simulink model "Integration_1.0"  (R2024b)
settings: Solver=VariableStepAuto  StartTime=0.0  StopTime=4  RelTol=1e-3
undefined symbols (not defined in the file): Ion, Lithium, Ts_Control
libraries: spsSeriesRLCBranchLib x37, ee_lib x30, nesl_utility x24, simulink x23, slpidlib x21, spsCurrentVoltageSimscapeInterfaceLib x18, powerlib_extras x18, spsThreePhaseVIMeasurementLib x7, spsThreePhaseSeriesRLCBranchLib x7, spsGroundLib x7, spsPWMGeneratorDCDCLib x6, spsPVArrayLib x6
(part 1 of 5)
settings Model: Creator=DELL  LastModifiedBy=mitphanase

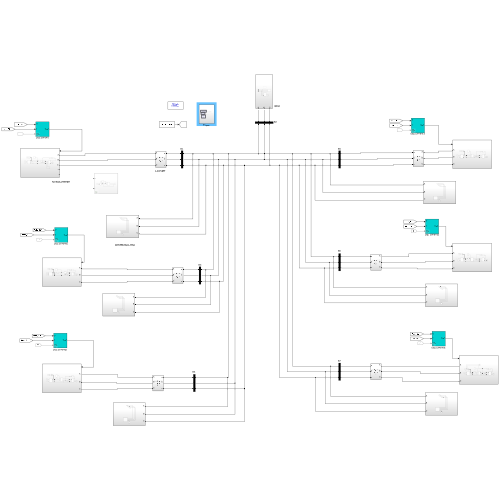
[thumbnail: Simulink's stored preview of the top-level diagram]
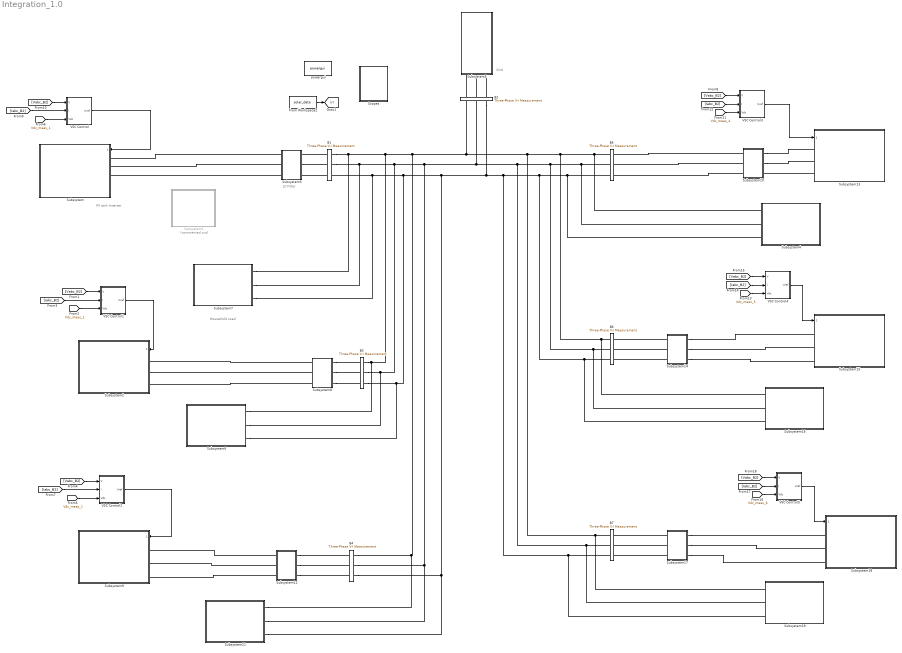
== system Integration_1.0 ==
  note: Household Load
  note: LC Filter
  note: Grid
  note: PV with Inverter
  B1 : spsThreePhaseVIMeasurementLib/Three-Phase V-I Measurement  VoltageMeasurement=phase-to-phase  SetLabelV=on  LabelV=Vabc_B1  Vpu=off  VpuLL=off  CurrentMeasurement=yes  SetLabelI=on  LabelI=Iabc_B1  Ipu=off  Pbase=100e6  Vbase=1000  OutputType=Magnitude  PhasorSimulation=off  PSBequivalent=0
  B2 : spsThreePhaseVIMeasurementLib/Three-Phase V-I Measurement  VoltageMeasurement=phase-to-phase  SetLabelV=on  LabelV=Vabc_B2  Vpu=off  VpuLL=off  CurrentMeasurement=yes  SetLabelI=on  LabelI=Iabc_B2  Ipu=off  Pbase=100e6  Vbase=500e3  OutputType=Magnitude  PhasorSimulation=off  PSBequivalent=0
  B3 : spsThreePhaseVIMeasurementLib/Three-Phase V-I Measurement  VoltageMeasurement=phase-to-phase  SetLabelV=on  LabelV=Vabc_B3  Vpu=off  VpuLL=off  CurrentMeasurement=yes  SetLabelI=on  LabelI=Iabc_B3  Ipu=off  Pbase=100e6  Vbase=1000  OutputType=Magnitude  PhasorSimulation=off  PSBequivalent=0
  B4 : spsThreePhaseVIMeasurementLib/Three-Phase V-I Measurement  VoltageMeasurement=phase-to-phase  SetLabelV=on  LabelV=Vabc_B4  Vpu=off  VpuLL=off  CurrentMeasurement=yes  SetLabelI=on  LabelI=Iabc_B4  Ipu=off  Pbase=100e6  Vbase=1000  OutputType=Magnitude  PhasorSimulation=off  PSBequivalent=0
  B5 : spsThreePhaseVIMeasurementLib/Three-Phase V-I Measurement  VoltageMeasurement=phase-to-phase  SetLabelV=on  LabelV=Vabc_B5  Vpu=off  VpuLL=off  CurrentMeasurement=yes  SetLabelI=on  LabelI=Iabc_B5  Ipu=off  Pbase=100e6  Vbase=1000  OutputType=Magnitude  PhasorSimulation=off  PSBequivalent=0
  B6 : spsThreePhaseVIMeasurementLib/Three-Phase V-I Measurement  VoltageMeasurement=phase-to-phase  SetLabelV=on  LabelV=Vabc_B6  Vpu=off  VpuLL=off  CurrentMeasurement=yes  SetLabelI=on  LabelI=Iabc_B6  Ipu=off  Pbase=100e6  Vbase=1000  OutputType=Magnitude  PhasorSimulation=off  PSBequivalent=0
  B7 : spsThreePhaseVIMeasurementLib/Three-Phase V-I Measurement  VoltageMeasurement=phase-to-phase  SetLabelV=on  LabelV=Vabc_B7  Vpu=off  VpuLL=off  CurrentMeasurement=yes  SetLabelI=on  LabelI=Iabc_B7  Ipu=off  Pbase=100e6  Vbase=1000  OutputType=Magnitude  PhasorSimulation=off  PSBequivalent=0
  From Workspace2 : FromWorkspace  VariableName=solar_data  OutDataTypeStr=double  SampleTime=0.01
  Scopes : Subsystem
  Subsystem : Subsystem
  Subsystem1 : Subsystem  Commented=on
  Subsystem10 : Subsystem
  Subsystem11 : Subsystem
  Subsystem12 : Subsystem
  Subsystem13 : Subsystem
  Subsystem14 : Subsystem
  Subsystem15 : Subsystem
  Subsystem16 : Subsystem
  Subsystem17 : Subsystem
  Subsystem18 : Subsystem
  Subsystem19 : Subsystem
  Subsystem2 : Subsystem
  Subsystem3 : Subsystem
  Subsystem4 : Subsystem
  Subsystem5 : Subsystem
  Subsystem6 : Subsystem
  Subsystem7 : Subsystem
  Subsystem8 : Subsystem
  Subsystem9 : Subsystem
  VSC Control : Subsystem  mask(VSC Main Controller){nom=[ 17e3  50 ], Vnom=[ 400 400 ], Vnom_dc=600, RLxfo=[0  0 ], RLchoke=[0  0  ], K_VDCreg=[18  600], K_Ireg=[0.2 20], Ts=Ts_Control}
      mask prompts: nom "Nominal power and frequency [ Pnom(VA)  Fnom(Hz) ]:"; Vnom "Nominal primary and secondary voltages (Vrms LL) [ Vnom_prim   Vnom_sec ]:"; Vnom_dc "Nominal DC bus voltage (V):"; RLxfo "Total transformer leakage impedance (pu/Pnom) [ Rxfo  Lxf ]"; RLchoke "Choke impedance [ R(ohm) L(H) ]"; K_VDCreg "VDC regultator gains [ Kp  Ki ]:"; K_Ireg "Current regulator gains [ Kp  Ki ]:"; Ts "Sample time"
      mask init:
      | Pnom=nom(1);
      | Fnom=nom(2);
      | Vnom_prim=Vnom(1);
      | Vnom_sec=Vnom(2);
      | Zbase=Vnom_sec^2/Pnom;
      | Rtot_pu=RLxfo(1) + RLchoke(1)/Zbase;
      | Ltot_pu=RLxfo(2) + RLchoke(2)/(Zbase/(2*pi*Fnom));
      | Kp_VDCreg=K_VDCreg(1);
      | Ki_VDCreg=K_VDCreg(2);
      | Kp_Ireg=K_Ireg(1);
      | Ki_Ireg=K_Ireg(2);
      | Vdc_ref=Vnom_dc;
  VSC Control1 : Subsystem  mask(VSC Main Controller){nom=[ 5e3  50 ], Vnom=[ 400 400 ], Vnom_dc=600, RLxfo=[0  0 ], RLchoke=[0  0  ], K_VDCreg=[18  600], K_Ireg=[0.2 20], Ts=Ts_Control}
      mask prompts: nom "Nominal power and frequency [ Pnom(VA)  Fnom(Hz) ]:"; Vnom "Nominal primary and secondary voltages (Vrms LL) [ Vnom_prim   Vnom_sec ]:"; Vnom_dc "Nominal DC bus voltage (V):"; RLxfo "Total transformer leakage impedance (pu/Pnom) [ Rxfo  Lxf ]"; RLchoke "Choke impedance [ R(ohm) L(H) ]"; K_VDCreg "VDC regultator gains [ Kp  Ki ]:"; K_Ireg "Current regulator gains [ Kp  Ki ]:"; Ts "Sample time"
      mask init: same as Integration_1.0/VSC Control
  VSC Control2 : Subsystem  mask(VSC Main Controller){nom=[ 5e3  50 ], Vnom=[ 400 400 ], Vnom_dc=600, RLxfo=[0  0 ], RLchoke=[0  0  ], K_VDCreg=[18  600], K_Ireg=[0.2 20], Ts=Ts_Control}
      mask prompts: nom "Nominal power and frequency [ Pnom(VA)  Fnom(Hz) ]:"; Vnom "Nominal primary and secondary voltages (Vrms LL) [ Vnom_prim   Vnom_sec ]:"; Vnom_dc "Nominal DC bus voltage (V):"; RLxfo "Total transformer leakage impedance (pu/Pnom) [ Rxfo  Lxf ]"; RLchoke "Choke impedance [ R(ohm) L(H) ]"; K_VDCreg "VDC regultator gains [ Kp  Ki ]:"; K_Ireg "Current regulator gains [ Kp  Ki ]:"; Ts "Sample time"
      mask init: same as Integration_1.0/VSC Control
  VSC Control3 : Subsystem  mask(VSC Main Controller){nom=[ 12.5e3  50 ], Vnom=[ 400 400 ], Vnom_dc=600, RLxfo=[0  0 ], RLchoke=[0  0  ], K_VDCreg=[18  600], K_Ireg=[0.2 20], Ts=Ts_Control}
      mask prompts: nom "Nominal power and frequency [ Pnom(VA)  Fnom(Hz) ]:"; Vnom "Nominal primary and secondary voltages (Vrms LL) [ Vnom_prim   Vnom_sec ]:"; Vnom_dc "Nominal DC bus voltage (V):"; RLxfo "Total transformer leakage impedance (pu/Pnom) [ Rxfo  Lxf ]"; RLchoke "Choke impedance [ R(ohm) L(H) ]"; K_VDCreg "VDC regultator gains [ Kp  Ki ]:"; K_Ireg "Current regulator gains [ Kp  Ki ]:"; Ts "Sample time"
      mask init: same as Integration_1.0/VSC Control
  VSC Control4 : Subsystem  mask(VSC Main Controller){nom=[ 8.5e3  50 ], Vnom=[ 400 400 ], Vnom_dc=600, RLxfo=[0  0 ], RLchoke=[0  0  ], K_VDCreg=[18  600], K_Ireg=[0.2 20], Ts=Ts_Control}
      mask prompts: nom "Nominal power and frequency [ Pnom(VA)  Fnom(Hz) ]:"; Vnom "Nominal primary and secondary voltages (Vrms LL) [ Vnom_prim   Vnom_sec ]:"; Vnom_dc "Nominal DC bus voltage (V):"; RLxfo "Total transformer leakage impedance (pu/Pnom) [ Rxfo  Lxf ]"; RLchoke "Choke impedance [ R(ohm) L(H) ]"; K_VDCreg "VDC regultator gains [ Kp  Ki ]:"; K_Ireg "Current regulator gains [ Kp  Ki ]:"; Ts "Sample time"
      mask init: same as Integration_1.0/VSC Control
  VSC Control5 : Subsystem  mask(VSC Main Controller){nom=[ 5e3  50 ], Vnom=[ 400 400 ], Vnom_dc=600, RLxfo=[0  0 ], RLchoke=[0  0  ], K_VDCreg=[18  600], K_Ireg=[0.2 20], Ts=Ts_Control}
      mask prompts: nom "Nominal power and frequency [ Pnom(VA)  Fnom(Hz) ]:"; Vnom "Nominal primary and secondary voltages (Vrms LL) [ Vnom_prim   Vnom_sec ]:"; Vnom_dc "Nominal DC bus voltage (V):"; RLxfo "Total transformer leakage impedance (pu/Pnom) [ Rxfo  Lxf ]"; RLchoke "Choke impedance [ R(ohm) L(H) ]"; K_VDCreg "VDC regultator gains [ Kp  Ki ]:"; K_Ireg "Current regulator gains [ Kp  Ki ]:"; Ts "Sample time"
      mask init: same as Integration_1.0/VSC Control
  powergui : sps_lib/powergui  Priority=1  SimulationMode=Discrete  SampleTime=5e-4  frequency=60  Iterations=50  frequencyindice=0  Pbase=100e6  ErrMax=1e-4  UnitsV=kV  UnitsW=MW  buscounter=0  FunctionMessages=off  echomessages=off  EnableUseOfTLC=off  CurrentSourceSwitches=off  DisableSnubberDevices=off  DisableRonSwitches=off  DisableVfSwitches=off  DisplayEquations=off  AutomaticDiscreteSolvers=off  SolverType=Tustin/Backward Euler (TBE)  Interpol=off  ExternalGateDelay=off  methode=off  Ts=100  x0status=blocks  SPID=on  SwTol=0  HookPort=off  NonlinearTolerance=1e-4  nMaxIteration=100  ContinueOnMaxIteration=off  RestoreLinks=warning  ResistiveCurrentMeasurement=off  Frange=[0:2:500]  Ylog=off  Xlog=on  ShowGrid=off  save=off  variable=ZData  structure=0  ZoomFFT=off  StartTime=0.0  cycles=1  DisplayStyle=1  fundamental=60  FreqAxis=off  MaxFrequency=1000  frequencyindicesteady=1  RmsSteady=1  display=off
  tag scope: irr=global
  wires:
  [Vdc_meas_1] -> VSC Control/3(Vdc)
  [Vabc_B2] -> VSC Control/1(V)
  [Iabc_B2] -> VSC Control/2(I)
  VSC Control/1(Uref) -> Subsystem/1("  ")
  From Workspace2/1 -> [irr]
  [Iabc_B2] -> VSC Control1/2(I)
  [Vabc_B2] -> VSC Control1/1(V)
  [Vdc_meas_1] -> VSC Control1/3(Vdc)
  VSC Control1/1(Uref) -> Subsystem2/1("  ")
  [Vabc_B2] -> VSC Control2/1(V)
  [Vdc_meas_1] -> VSC Control2/3(Vdc)
  [Iabc_B2] -> VSC Control2/2(I)
  VSC Control2/1(Uref) -> Subsystem9/1("  ")
  VSC Control3/1(Uref) -> Subsystem13/1("  ")
  [Vabc_B2] -> VSC Control3/1(V)
  [Iabc_B2] -> VSC Control3/2(I)
  [Vdc_meas_4] -> VSC Control3/3(Vdc)
  [Vdc_meas_5] -> VSC Control4/3(Vdc)
  [Iabc_B2] -> VSC Control4/2(I)
  [Vabc_B2] -> VSC Control4/1(V)
  VSC Control4/1(Uref) -> Subsystem15/1("  ")
  VSC Control5/1(Uref) -> Subsystem18/1("  ")
  [Vabc_B2] -> VSC Control5/1(V)
  [Iabc_B2] -> VSC Control5/2(I)
  [Vdc_meas_6] -> VSC Control5/3(Vdc)
  connections:
  B1/RConn1 -- Subsystem7/LConn1 -- Subsystem6/LConn1 -- B3/RConn1 -- Subsystem11/LConn1 -- B4/RConn1 -- Subsystem19/LConn1 -- B7/RConn1 -- Subsystem16/LConn1 -- B6/RConn1 -- Subsystem4/LConn1 -- B5/RConn1 -- B2/RConn1
  B2/RConn3 -- Subsystem11/LConn3 -- B4/RConn3 -- Subsystem6/LConn3 -- B3/RConn3 -- Subsystem7/LConn3 -- B1/RConn3 -- Subsystem19/LConn3 -- B7/RConn3 -- Subsystem16/LConn3 -- B6/RConn3 -- Subsystem4/LConn3 -- B5/RConn3
  B1/RConn2 -- Subsystem7/LConn2 -- Subsystem6/LConn2 -- B3/RConn2 -- Subsystem11/LConn2 -- B4/RConn2 -- Subsystem19/LConn2 -- B7/RConn2 -- Subsystem16/LConn2 -- B6/RConn2 -- Subsystem4/LConn2 -- B5/RConn2 -- B2/RConn2
  B1/LConn3 -- Subsystem3/RConn3
  B1/LConn1 -- Subsystem3/RConn1
  B1/LConn2 -- Subsystem3/RConn2
  Subsystem3/LConn1 -- Subsystem/LConn1
  Subsystem3/LConn2 -- Subsystem/LConn2
  Subsystem3/LConn3 -- Subsystem/LConn3
  B2/LConn1 -- Subsystem5/LConn1
  B2/LConn2 -- Subsystem5/LConn2
  B2/LConn3 -- Subsystem5/LConn3
  Subsystem12/RConn1 -- B4/LConn1
  Subsystem12/LConn2 -- Subsystem9/LConn2
  Subsystem12/RConn3 -- B4/LConn3
  Subsystem12/LConn3 -- Subsystem9/LConn3
  Subsystem12/LConn1 -- Subsystem9/LConn1
  Subsystem12/RConn2 -- B4/LConn2
  Subsystem14/LConn2 -- Subsystem15/LConn2
  Subsystem14/RConn3 -- B6/LConn3
  Subsystem14/LConn1 -- Subsystem15/LConn1
  Subsystem14/LConn3 -- Subsystem15/LConn3
  Subsystem14/RConn1 -- B6/LConn1
  Subsystem14/RConn2 -- B6/LConn2
  Subsystem17/LConn2 -- Subsystem18/LConn2
  Subsystem17/RConn3 -- B7/LConn3
  Subsystem17/LConn1 -- Subsystem18/LConn1
  Subsystem17/LConn3 -- Subsystem18/LConn3
  Subsystem17/RConn1 -- B7/LConn1
  Subsystem17/RConn2 -- B7/LConn2
  Subsystem8/RConn1 -- B3/LConn1
  Subsystem8/RConn2 -- B3/LConn2
  Subsystem8/RConn3 -- B3/LConn3
  Subsystem8/LConn1 -- Subsystem2/LConn1
  Subsystem8/LConn2 -- Subsystem2/LConn2
  Subsystem8/LConn3 -- Subsystem2/LConn3
  Subsystem10/RConn1 -- B5/LConn1
  Subsystem10/RConn2 -- B5/LConn2
  Subsystem10/RConn3 -- B5/LConn3
  Subsystem10/LConn2 -- Subsystem13/LConn2
  Subsystem10/LConn1 -- Subsystem13/LConn1
  Subsystem13/LConn3 -- Subsystem10/LConn3

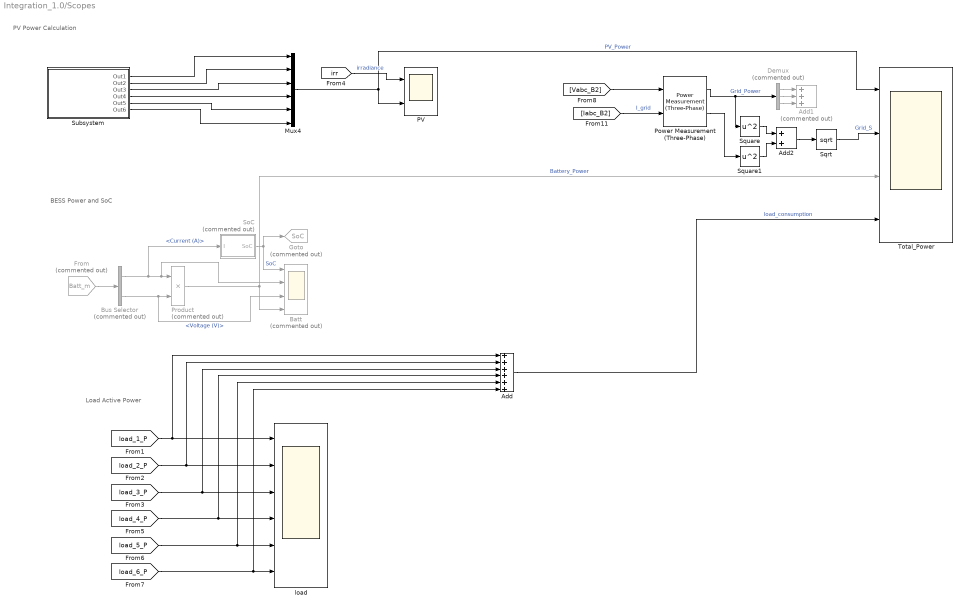
== system Integration_1.0/Scopes ==
  note: Load Active Power
  note: BESS Power and SoC
  note: PV Power Calculation
  Add : Sum  Inputs=++++++
  Add1 : Sum  Commented=on  Inputs=+++
  Add2 : Sum
  Batt : Scope  Commented=on  NumInputPorts=4
  Bus Selector : BusSelector  Commented=on  OutputSignals=Current (A),Voltage (V)
  Demux : Demux  Commented=on  Outputs=3
  From : From  Commented=on  GotoTag=Batt_m  TagVisibility=global
  Goto : Goto  Commented=on  GotoTag=SoC  TagVisibility=global
  Mux4 : Mux  Inputs=6
  PV : Scope  NumInputPorts=2
  Power Measurement (Three-Phase) : eePowerMeasurement/Power Measurement (Three-Phase)  LabelModeActiveChoice=Discrete  F=50  K=[0 1 3 5]  Seq=Positive  Ts=Ts_Control
  Product : Product  Commented=on
  SoC : Subsystem  Commented=on
  Sqrt : Sqrt
  Square : Math  Operator=square
  Square1 : Math  Operator=square
  Subsystem : Subsystem
  Total_Power : Scope  NumInputPorts=4
  load : Scope  NumInputPorts=6
  wires:
  [irr] -> PV/1  "irradiance"
  SoC/1(SoC) -> Goto/1, Batt/1  "SoC"
  Subsystem/1(Out1) -> Mux4/1
  Subsystem/2(Out2) -> Mux4/2
  Subsystem/3(Out3) -> Mux4/3
  Subsystem/4(Out4) -> Mux4/4
  Subsystem/5(Out5) -> Mux4/5
  Subsystem/6(Out6) -> Mux4/6
  Mux4/1 -> Total_Power/1, PV/2  "PV_Power"
  From/1 -> Bus Selector/1
  Bus Selector/1 -> SoC/1(I), Batt/2, Product/1  "<Current (A)>"
  Bus Selector/2 -> Batt/3, Product/2  "<Voltage (V)>"
  Product/1 -> Total_Power/3, Batt/4  "Battery_Power"
  [load_1_P] -> Add/1, load/1
  [load_4_P] -> Add/4, load/4
  [load_3_P] -> Add/3, load/3
  [load_2_P] -> Add/2, load/2
  [load_5_P] -> Add/5, load/5
  [load_6_P] -> Add/6, load/6
  [Vabc_B2] -> Power Measurement (Three-Phase)/1
  [Iabc_B2] -> Power Measurement (Three-Phase)/2  "I_grid"
  Power Measurement (Three-Phase)/1 -> Square/1, Demux/1  "Grid_Power"
  Add/1 -> Total_Power/4  "load_consumption"
  Demux/1 -> Add1/1
  Demux/2 -> Add1/2
  Demux/3 -> Add1/3
  Power Measurement (Three-Phase)/2 -> Square1/1
  Square/1 -> Add2/1
  Square1/1 -> Add2/2
  Add2/1 -> Sqrt/1
  Sqrt/1 -> Total_Power/2  "Grid_S"

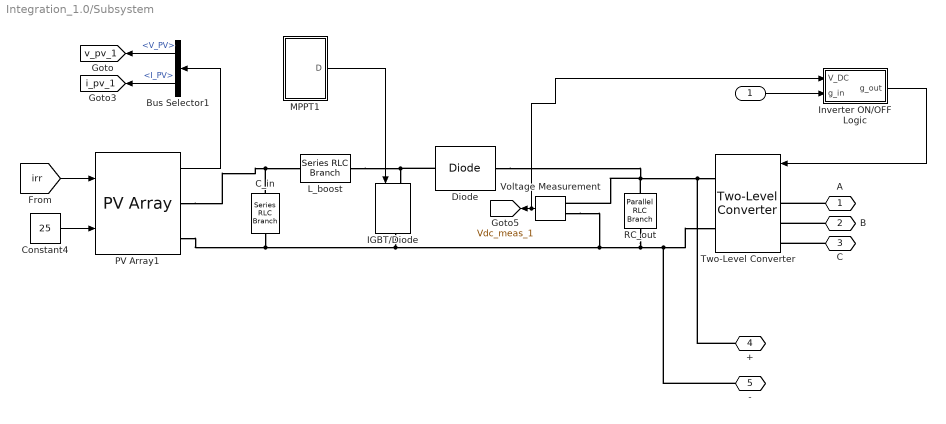
== system Integration_1.0/Subsystem ==
  "  " : Inport
  Bus Selector1 : BusSelector  OutputSignals=V_PV,I_PV
  C_in : spsSeriesRLCBranchLib/Series RLC Branch  LConnTagsString=__new0  RConnTagsString=__new0  BranchType=C  Resistance=1e-5  Inductance=1e-3  SetiL0=off  InitialCurrent=0  Capacitance=850e-6  Setx0=off  InitialVoltage=426.5  Measurements=Branch voltage and current
  Constant4 : Constant  Value=25
  Diode : spsDiodeLib/Diode  Ron=0.001  Lon=0  Vf=0.8  IC=0  UseSnubber=0  Rs=500  Cs=250e-9  Measurements=off
  IGBT/Diode : spsIGBTDiodeLib/IGBT//Diode  Ron=1e-3  Rs=1e5  Cs=inf  Measurements=off
  Inverter ON/OFF Logic : Subsystem
  L_boost : spsSeriesRLCBranchLib/Series RLC Branch  LConnTagsString=__new0  RConnTagsString=__new0  BranchType=L  Resistance=1e-3  Inductance=58e-3  SetiL0=off  InitialCurrent=0  Capacitance=100e-6  Setx0=off  InitialVoltage=230  Measurements=None
  MPPT1 : Subsystem
  PV Array1 : spsPVArrayLib/PV Array  Npar=8  Nser=5  PlotType=array @ 1000 W/m2 & specified temperatures  S_vec="[ 1000  500  100 ]"  Temp_C_vec="[ 45 25  ]"  ModuleName=SunPower SPR-415E-WHT-D  PlotWhenSelected=off  Pm=414.801  Ncell=128  Voc=85.3  Isc=6.09  Vm=72.9  Im=5.69  beta_Voc_pc=-0.229  alpha_Isc_pc=0.030706  beta_Voc=-0.19534  alpha_Isc=0.00187  IL=6.0978  I0=7.1698e-13  nI=0.87223  Rsh=419.7781  Rs=0.53711  RobustModel=off  RobustCellTemperature=313.3991  BAL=on  Tc=1e-6  Tfilter=5e-5
  RC_out : spsParallelRLCBranchLib/Parallel RLC Branch  LConnTagsString=a  RConnTagsString=__new0  BranchType=C  Resistance=20  Inductance=1e-3  SetiL0=off  InitialCurrent=0  Capacitance=5*636e-6  Setx0=off  InitialVoltage=700  Measurements=None
  Two-Level Converter : spsTwoLevelConverterLib/Two-Level Converter  ModelType=Average model (Uref-controlled)  Ron=1e-3  Rs=1e6  Cs=inf  Vforward=[0,0]  Ron_Diode=1e-3  Rs_Diode=1e6  Cs_Diode=inf  Vf_Diode=1e-3  Rs_CurrentSource=inf  Ron_ACsource=1e-3
      settings: LibrarySourceBlock=sps_lib/Power Electronics/Two-Level Converter
  Voltage Measurement : spsVoltageMeasurementLib/Voltage Measurement  PhasorSimulation=off  OutputType=Complex  PSBequivalent=0
  A : PMIOPort  Side=Left
  B : PMIOPort  Port=2  Side=Left
  C : PMIOPort  Port=3  Side=Left
  + : PMIOPort  Port=4  Side=Left
  - : PMIOPort  Port=5  Side=Left
  tag scope: Vdc_meas_1=global, i_pv_1=global, v_pv_1=global
  wires:
  Voltage Measurement/1 -> Inverter ON/OFF Logic/1(V_DC), [Vdc_meas_1]
  Bus Selector1/1 -> [v_pv_1]  "<V_PV>"
  Constant4/1 -> PV Array1/2
  Bus Selector1/2 -> [i_pv_1]  "<I_PV>"
  PV Array1/1 -> Bus Selector1/1
  [irr] -> PV Array1/1
  MPPT1/1(D) -> IGBT/Diode/1
  "  "/1 -> Inverter ON/OFF Logic/2(g_in)
  Inverter ON/OFF Logic/1(g_out) -> Two-Level Converter/1
  connections:
  A/RConn1 -- Two-Level Converter/LConn1
  PV Array1/RConn2 -- C_in/RConn1 -- Voltage Measurement/LConn2 -- RC_out/RConn1 -- -/RConn1 -- Two-Level Converter/RConn2 -- IGBT/Diode/RConn1
  PV Array1/RConn1 -- C_in/LConn1 -- L_boost/LConn1
  Voltage Measurement/LConn1 -- Diode/RConn1 -- RC_out/LConn1 -- +/RConn1 -- Two-Level Converter/RConn1
  C/RConn1 -- Two-Level Converter/LConn3
  B/RConn1 -- Two-Level Converter/LConn2
  L_boost/RConn1 -- Diode/LConn1 -- IGBT/Diode/LConn1

== system Integration_1.0/Subsystem1 ==
  BATT chg-dshg logic1 : Subsystem
  Battery : spsBatteryLib/Battery  BatType=Lithium-Ion  NomV=48  NomQ=100  SOC=0  Batt_Tr=46.3e-3  PresetModel=on  MaxQ=100  MinV=36  FullV=55.8714  Dis_rate=43.4783  R=0.0048  Normal_OP=90.4348  expZone="[51.8585      4.91304]"
  Current Measurement : spsCurrentMeasurementLib/Current Measurement  PhasorSimulation=off  OutputType=Complex  PSBequivalent=0
  L_B : spsSeriesRLCBranchLib/Series RLC Branch  LConnTagsString=__new0  RConnTagsString=__new0  BranchType=L  Resistance=1e-3  Inductance=5e-3  SetiL0=off  InitialCurrent=0  Capacitance=100e-6  Setx0=off  InitialVoltage=230  Measurements=None
  Two-Quadrant DC/DC Converter : spsTwoQuadrantDCDCConverterLib/Two-Quadrant DC//DC Converter  ModelType=Average model (D-controlled)  Ron=1e-3  Rs=1e6  Cs=inf  Vforward=[0,0]  Ron_Diode=1e-3  Rs_Diode=1e6  Cs_Diode=inf  Vf_Diode=1e-3  Rs_CurrentSource=inf  Ron_ACsource=1e-3
  + : PMIOPort  Side=Left
  - : PMIOPort  Port=2  Side=Left
  tag scope: Batt_m=global
  wires:
  BATT chg-dshg logic1/1(D) -> Two-Quadrant DC/DC Converter/1
  Battery/1 -> [Batt_m]
  Current Measurement/1 -> BATT chg-dshg logic1/1(I_B)
  connections:
  Two-Quadrant DC/DC Converter/RConn1 -- +/RConn1
  Battery/LConn2 -- Two-Quadrant DC/DC Converter/RConn2 -- -/RConn1
  L_B/RConn1 -- Two-Quadrant DC/DC Converter/LConn1
  Current Measurement/RConn1 -- Battery/LConn1
  Current Measurement/LConn1 -- L_B/LConn1

== system Integration_1.0/Subsystem10 ==
  Series RLC Branch1 : spsSeriesRLCBranchLib/Series RLC Branch  LConnTagsString=__new0  RConnTagsString=__new0  BranchType=C  Resistance=10  Inductance=1e-3  SetiL0=off  InitialCurrent=0  Capacitance=0.81e-6  Setx0=off  InitialVoltage=0  Measurements=None
  Series RLC Branch2 : spsSeriesRLCBranchLib/Series RLC Branch  LConnTagsString=__new0  RConnTagsString=__new0  BranchType=C  Resistance=10  Inductance=1e-3  SetiL0=off  InitialCurrent=0  Capacitance=0.81e-6  Setx0=off  InitialVoltage=0  Measurements=None
  Series RLC Branch3 : spsSeriesRLCBranchLib/Series RLC Branch  LConnTagsString=__new0  RConnTagsString=__new0  BranchType=C  Resistance=10  Inductance=1e-3  SetiL0=off  InitialCurrent=0  Capacitance=0.81e-6  Setx0=off  InitialVoltage=0  Measurements=None
  Three-Phase Series RLC Branch1 : spsThreePhaseSeriesRLCBranchLib/Three-Phase Series RLC Branch  LConnTagsString=A|B|C  RConnTagsString=A|B|C  BranchType=L  Resistance=1  Inductance=3*7.42e-3  Capacitance=1e-6  Measurements=None
  A : PMIOPort  Side=Left
  B : PMIOPort  Port=2  Side=Left
  C : PMIOPort  Port=3  Side=Left
  a : PMIOPort  Port=4  Side=Right
  b : PMIOPort  Port=5  Side=Right
  c : PMIOPort  Port=6  Side=Right
  connections:
  c/RConn1 -- Three-Phase Series RLC Branch1/RConn3 -- Series RLC Branch2/LConn1 -- Series RLC Branch1/RConn1
  Three-Phase Series RLC Branch1/LConn3 -- C/RConn1
  Three-Phase Series RLC Branch1/LConn2 -- B/RConn1
  Three-Phase Series RLC Branch1/LConn1 -- A/RConn1
  a/RConn1 -- Three-Phase Series RLC Branch1/RConn1 -- Series RLC Branch3/LConn1 -- Series RLC Branch2/RConn1
  b/RConn1 -- Series RLC Branch3/RConn1 -- Series RLC Branch1/LConn1 -- Three-Phase Series RLC Branch1/RConn2

== system Integration_1.0/Subsystem11 ==
  Ground1 : spsGroundLib/Ground  LConnTagsString=a
  Subsystem2 : Subsystem
  A : PMIOPort  Side=Left
  B : PMIOPort  Port=2  Side=Left
  C : PMIOPort  Port=3  Side=Left
  connections:
  Subsystem2/LConn2 -- B/RConn1
  Subsystem2/LConn4 -- Ground1/LConn1
  Subsystem2/LConn1 -- A/RConn1
  Subsystem2/LConn3 -- C/RConn1

== system Integration_1.0/Subsystem12 ==
  Series RLC Branch1 : spsSeriesRLCBranchLib/Series RLC Branch  LConnTagsString=__new0  RConnTagsString=__new0  BranchType=C  Resistance=5  Inductance=1e-3  SetiL0=off  InitialCurrent=0  Capacitance=0.41e-6  Setx0=off  InitialVoltage=0  Measurements=None
  Series RLC Branch2 : spsSeriesRLCBranchLib/Series RLC Branch  LConnTagsString=__new0  RConnTagsString=__new0  BranchType=C  Resistance=5  Inductance=1e-3  SetiL0=off  InitialCurrent=0  Capacitance=0.41e-6  Setx0=off  InitialVoltage=0  Measurements=None
  Series RLC Branch3 : spsSeriesRLCBranchLib/Series RLC Branch  LConnTagsString=__new0  RConnTagsString=__new0  BranchType=C  Resistance=5  Inductance=1e-3  SetiL0=off  InitialCurrent=0  Capacitance=0.41e-6  Setx0=off  InitialVoltage=0  Measurements=None
  Three-Phase Series RLC Branch1 : spsThreePhaseSeriesRLCBranchLib/Three-Phase Series RLC Branch  LConnTagsString=A|B|C  RConnTagsString=A|B|C  BranchType=L  Resistance=1  Inductance=7.423e-3  Capacitance=1e-6  Measurements=None
  A : PMIOPort  Side=Left
  B : PMIOPort  Port=2  Side=Left
  C : PMIOPort  Port=3  Side=Left
  a : PMIOPort  Port=4  Side=Right
  b : PMIOPort  Port=5  Side=Right
  c : PMIOPort  Port=6  Side=Right
  connections:
  Three-Phase Series RLC Branch1/RConn2 -- Series RLC Branch1/LConn1 -- Series RLC Branch3/RConn1 -- b/RConn1
  Series RLC Branch2/RConn1 -- Series RLC Branch3/LConn1 -- Three-Phase Series RLC Branch1/RConn1 -- a/RConn1
  Three-Phase Series RLC Branch1/LConn1 -- A/RConn1
  Three-Phase Series RLC Branch1/LConn2 -- B/RConn1
  Three-Phase Series RLC Branch1/LConn3 -- C/RConn1
  Series RLC Branch1/RConn1 -- Series RLC Branch2/LConn1 -- Three-Phase Series RLC Branch1/RConn3 -- c/RConn1

== system Integration_1.0/Subsystem13 ==
  "  " : Inport
  Boost Converter : spsBoostConverterLib/Boost Converter  ModelType=Average model (D-controlled)  Ron=1e-3  Rs=1e6  Cs=inf  Vforward=[0,0]  Ron_Diode=1e-3  Rs_Diode=1e6  Cs_Diode=inf  Vf_Diode=1e-3  Rs_CurrentSource=inf  Ron_ACsource=1e-3
      settings: LibrarySourceBlock=sps_lib/Power Electronics/Boost Converter
  Bus Selector1 : BusSelector  OutputSignals=V_PV,I_PV
  C_in : spsSeriesRLCBranchLib/Series RLC Branch  LConnTagsString=__new0  RConnTagsString=__new0  BranchType=C  Resistance=1e-5  Inductance=1e-3  SetiL0=off  InitialCurrent=0  Capacitance=628.37e-6  Setx0=off  InitialVoltage=426.5  Measurements=None
  Constant4 : Constant  Value=25
  Inverter ON/OFF Logic : Subsystem
  L_boost : spsSeriesRLCBranchLib/Series RLC Branch  LConnTagsString=__new0  RConnTagsString=__new0  BranchType=L  Resistance=1e-3  Inductance=78.31e-3  SetiL0=off  InitialCurrent=0  Capacitance=100e-6  Setx0=off  InitialVoltage=230  Measurements=None
  MPPT1 : Subsystem
  PV Array1 : spsPVArrayLib/PV Array  Npar=6  Nser=5  PlotType=array @ 1000 W/m2 & specified temperatures  S_vec="[ 1000  500  100 ]"  Temp_C_vec="[ 45 25  ]"  ModuleName=SunPower SPR-415E-WHT-D  PlotWhenSelected=off  Pm=414.801  Ncell=128  Voc=85.3  Isc=6.09  Vm=72.9  Im=5.69  beta_Voc_pc=-0.229  alpha_Isc_pc=0.030706  beta_Voc=-0.19534  alpha_Isc=0.00187  IL=6.0978  I0=7.1698e-13  nI=0.87223  Rsh=419.7781  Rs=0.53711  RobustModel=off  RobustCellTemperature=313.3991  BAL=on  Tc=1e-6  Tfilter=5e-5
  RC_out : spsParallelRLCBranchLib/Parallel RLC Branch  LConnTagsString=a  RConnTagsString=__new0  BranchType=C  Resistance=5  Inductance=1e-3  SetiL0=off  InitialCurrent=0  Capacitance=5*478.065e-6  Setx0=off  InitialVoltage=700  Measurements=None
  Two-Level Converter : spsTwoLevelConverterLib/Two-Level Converter  ModelType=Average model (No rectifier mode)  Ron=1e-3  Rs=1e6  Cs=inf  Vforward=[0,0]  Ron_Diode=1e-3  Rs_Diode=1e6  Cs_Diode=inf  Vf_Diode=1e-3  Rs_CurrentSource=inf  Ron_ACsource=1e-3
  Voltage Measurement : spsVoltageMeasurementLib/Voltage Measurement  PhasorSimulation=off  OutputType=Complex  PSBequivalent=0
  A : PMIOPort  Side=Left
  B : PMIOPort  Port=2  Side=Left
  C : PMIOPort  Port=3  Side=Left
  tag scope: Vdc_meas_4=global, i_pv_4=global, v_pv_4=global
  wires:
  Voltage Measurement/1 -> Inverter ON/OFF Logic/1(V_DC), [Vdc_meas_4]
  Bus Selector1/1 -> [v_pv_4]  "<V_PV>"
  Constant4/1 -> PV Array1/2
  Bus Selector1/2 -> [i_pv_4]  "<I_PV>"
  PV Array1/1 -> Bus Selector1/1
  [irr] -> PV Array1/1
  MPPT1/1(D) -> Boost Converter/1
  Inverter ON/OFF Logic/1(g_out) -> Two-Level Converter/1
  "  "/1 -> Inverter ON/OFF Logic/2(g_in)
  connections:
  A/RConn1 -- Two-Level Converter/LConn1
  Two-Level Converter/RConn2 -- RC_out/RConn1 -- Boost Converter/RConn2 -- C_in/RConn1 -- PV Array1/RConn2 -- Voltage Measurement/LConn2
  C_in/LConn1 -- L_boost/LConn1 -- PV Array1/RConn1
  RC_out/LConn1 -- Boost Converter/RConn1 -- Voltage Measurement/LConn1 -- Two-Level Converter/RConn1
  C/RConn1 -- Two-Level Converter/LConn3
  B/RConn1 -- Two-Level Converter/LConn2
  L_boost/RConn1 -- Boost Converter/LConn1

== system Integration_1.0/Subsystem14 ==
  Series RLC Branch1 : spsSeriesRLCBranchLib/Series RLC Branch  LConnTagsString=__new0  RConnTagsString=__new0  BranchType=RC  Resistance=10  Inductance=1e-3  SetiL0=off  InitialCurrent=0  Capacitance=3*15e-6  Setx0=off  InitialVoltage=0  Measurements=None
  Series RLC Branch2 : spsSeriesRLCBranchLib/Series RLC Branch  LConnTagsString=__new0  RConnTagsString=__new0  BranchType=RC  Resistance=10  Inductance=1e-3  SetiL0=off  InitialCurrent=0  Capacitance=3*15e-6  Setx0=off  InitialVoltage=0  Measurements=None
  Series RLC Branch3 : spsSeriesRLCBranchLib/Series RLC Branch  LConnTagsString=__new0  RConnTagsString=__new0  BranchType=RC  Resistance=10  Inductance=1e-3  SetiL0=off  InitialCurrent=0  Capacitance=3*15e-6  Setx0=off  InitialVoltage=0  Measurements=None
  Three-Phase Series RLC Branch1 : spsThreePhaseSeriesRLCBranchLib/Three-Phase Series RLC Branch  LConnTagsString=A|B|C  RConnTagsString=A|B|C  BranchType=L  Resistance=1  Inductance=3*6e-3  Capacitance=1e-6  Measurements=None
  Three-Phase Breaker : spsThreePhaseBreakerLib/Three-Phase Breaker  InitialState=closed  SwitchA=on  SwitchB=on  SwitchC=on  SwitchTimes="[1/60  5/60]"  External=off  BreakerResistance=0.01  SnubberResistance=1e6  SnubberCapacitance=inf  Measurements=None
  A : PMIOPort  Side=Left
  B : PMIOPort  Port=2  Side=Left
  C : PMIOPort  Port=3  Side=Left
  a : PMIOPort  Port=4  Side=Right
  b : PMIOPort  Port=5  Side=Right
  c : PMIOPort  Port=6  Side=Right
  connections:
  Series RLC Branch1/LConn1 -- Three-Phase Series RLC Branch1/RConn2 -- Three-Phase Breaker/LConn2 -- Series RLC Branch3/RConn1
  Series RLC Branch1/RConn1 -- Three-Phase Breaker/LConn3 -- Three-Phase Series RLC Branch1/RConn3 -- Series RLC Branch2/RConn1
  Series RLC Branch3/LConn1 -- Three-Phase Series RLC Branch1/RConn1 -- Three-Phase Breaker/LConn1 -- Series RLC Branch2/LConn1
  Three-Phase Series RLC Branch1/LConn1 -- A/RConn1
  Three-Phase Series RLC Branch1/LConn2 -- B/RConn1
  Three-Phase Series RLC Branch1/LConn3 -- C/RConn1
  Three-Phase Breaker/RConn1 -- a/RConn1
  b/RConn1 -- Three-Phase Breaker/RConn2
  c/RConn1 -- Three-Phase Breaker/RConn3

== system Integration_1.0/Subsystem15 ==
  "  " : Inport
  Boost Converter : spsBoostConverterLib/Boost Converter  ModelType=Average model (D-controlled)  Ron=1e-3  Rs=1e6  Cs=inf  Vforward=[0,0]  Ron_Diode=1e-3  Rs_Diode=1e6  Cs_Diode=inf  Vf_Diode=1e-3  Rs_CurrentSource=inf  Ron_ACsource=1e-3
      settings: LibrarySourceBlock=sps_lib/Power Electronics/Boost Converter
  Bus Selector1 : BusSelector  OutputSignals=V_PV,I_PV
  C_in : spsSeriesRLCBranchLib/Series RLC Branch  LConnTagsString=__new0  RConnTagsString=__new0  BranchType=C  Resistance=1e-5  Inductance=1e-3  SetiL0=off  InitialCurrent=0  Capacitance=418e-6  Setx0=off  InitialVoltage=426.5  Measurements=Branch voltage and current
  Constant4 : Constant  Value=25
  Inverter ON/OFF Logic : Subsystem
  L_boost : spsSeriesRLCBranchLib/Series RLC Branch  LConnTagsString=__new0  RConnTagsString=__new0  BranchType=L  Resistance=1e-3  Inductance=117.45e-3  SetiL0=off  InitialCurrent=0  Capacitance=100e-6  Setx0=off  InitialVoltage=230  Measurements=None
  MPPT1 : Subsystem
  PV Array1 : spsPVArrayLib/PV Array  Npar=5  Nser=4  PlotType=array @ 1000 W/m2 & specified temperatures  S_vec="[ 1000  500  100 ]"  Temp_C_vec="[ 45 25  ]"  ModuleName=SunPower SPR-415E-WHT-D  PlotWhenSelected=off  Pm=414.801  Ncell=128  Voc=85.3  Isc=6.09  Vm=72.9  Im=5.69  beta_Voc_pc=-0.229  alpha_Isc_pc=0.030706  beta_Voc=-0.19534  alpha_Isc=0.00187  IL=6.0978  I0=7.1698e-13  nI=0.87223  Rsh=419.7781  Rs=0.53711  RobustModel=off  RobustCellTemperature=313.3991  BAL=on  Tc=1e-6  Tfilter=5e-5
  RC_out : spsParallelRLCBranchLib/Parallel RLC Branch  LConnTagsString=a  RConnTagsString=__new0  BranchType=C  Resistance=5  Inductance=1e-3  SetiL0=off  InitialCurrent=0  Capacitance=5*318.7e-6  Setx0=off  InitialVoltage=700  Measurements=None
  Two-Level Converter : spsTwoLevelConverterLib/Two-Level Converter  ModelType=Average model (No rectifier mode)  Ron=1e-3  Rs=1e6  Cs=inf  Vforward=[0,0]  Ron_Diode=1e-3  Rs_Diode=1e6  Cs_Diode=inf  Vf_Diode=1e-3  Rs_CurrentSource=inf  Ron_ACsource=1e-3
  Voltage Measurement : spsVoltageMeasurementLib/Voltage Measurement  PhasorSimulation=off  OutputType=Complex  PSBequivalent=0
  A : PMIOPort  Side=Left
  B : PMIOPort  Port=2  Side=Left
  C : PMIOPort  Port=3  Side=Left
  tag scope: Vdc_meas_5=global, i_pv_5=global, v_pv_5=global
  wires:
  Bus Selector1/1 -> [v_pv_5]  "<V_PV>"
  Constant4/1 -> PV Array1/2
  Bus Selector1/2 -> [i_pv_5]  "<I_PV>"
  PV Array1/1 -> Bus Selector1/1
  [irr] -> PV Array1/1
  Voltage Measurement/1 -> Inverter ON/OFF Logic/1(V_DC), [Vdc_meas_5]
  Inverter ON/OFF Logic/1(g_out) -> Two-Level Converter/1
  "  "/1 -> Inverter ON/OFF Logic/2(g_in)
  MPPT1/1(D) -> Boost Converter/1
  connections:
  A/RConn1 -- Two-Level Converter/LConn1
  Two-Level Converter/RConn2 -- RC_out/RConn1 -- Voltage Measurement/LConn2 -- Boost Converter/RConn2 -- C_in/RConn1 -- PV Array1/RConn2
  C_in/LConn1 -- L_boost/LConn1 -- PV Array1/RConn1
  RC_out/LConn1 -- Boost Converter/RConn1 -- Voltage Measurement/LConn1 -- Two-Level Converter/RConn1
  C/RConn1 -- Two-Level Converter/LConn3
  B/RConn1 -- Two-Level Converter/LConn2
  Boost Converter/LConn1 -- L_boost/RConn1

== system Integration_1.0/Subsystem16 ==
  Ground1 : spsGroundLib/Ground  LConnTagsString=a
  Subsystem2 : Subsystem
  A : PMIOPort  Side=Left
  B : PMIOPort  Port=2  Side=Left
  C : PMIOPort  Port=3  Side=Left
  connections:
  Subsystem2/LConn2 -- B/RConn1
  Subsystem2/LConn4 -- Ground1/LConn1
  Subsystem2/LConn1 -- A/RConn1
  Subsystem2/LConn3 -- C/RConn1

== system Integration_1.0/Subsystem17 ==
  Series RLC Branch1 : spsSeriesRLCBranchLib/Series RLC Branch  LConnTagsString=__new0  RConnTagsString=__new0  BranchType=C  Resistance=10  Inductance=1e-3  SetiL0=off  InitialCurrent=0  Capacitance=0.54e-6  Setx0=off  InitialVoltage=0  Measurements=None
  Series RLC Branch2 : spsSeriesRLCBranchLib/Series RLC Branch  LConnTagsString=__new0  RConnTagsString=__new0  BranchType=C  Resistance=10  Inductance=1e-3  SetiL0=off  InitialCurrent=0  Capacitance=0.54e-6  Setx0=off  InitialVoltage=0  Measurements=None
  Series RLC Branch3 : spsSeriesRLCBranchLib/Series RLC Branch  LConnTagsString=__new0  RConnTagsString=__new0  BranchType=C  Resistance=10  Inductance=1e-3  SetiL0=off  InitialCurrent=0  Capacitance=0.54e-6  Setx0=off  InitialVoltage=0  Measurements=None
  Three-Phase Series RLC Branch1 : spsThreePhaseSeriesRLCBranchLib/Three-Phase Series RLC Branch  LConnTagsString=A|B|C  RConnTagsString=A|B|C  BranchType=L  Resistance=1  Inductance=3*5.56e-3  Capacitance=1e-6  Measurements=None
  A : PMIOPort  Side=Left
  B : PMIOPort  Port=2  Side=Left
  C : PMIOPort  Port=3  Side=Left
  a : PMIOPort  Port=4  Side=Right
  b : PMIOPort  Port=5  Side=Right
  c : PMIOPort  Port=6  Side=Right
  connections:
  c/RConn1 -- Three-Phase Series RLC Branch1/RConn3 -- Series RLC Branch2/LConn1 -- Series RLC Branch1/RConn1
  Three-Phase Series RLC Branch1/LConn3 -- C/RConn1
  Three-Phase Series RLC Branch1/LConn2 -- B/RConn1
  Three-Phase Series RLC Branch1/LConn1 -- A/RConn1
  a/RConn1 -- Three-Phase Series RLC Branch1/RConn1 -- Series RLC Branch3/LConn1 -- Series RLC Branch2/RConn1
  b/RConn1 -- Series RLC Branch3/RConn1 -- Series RLC Branch1/LConn1 -- Three-Phase Series RLC Branch1/RConn2

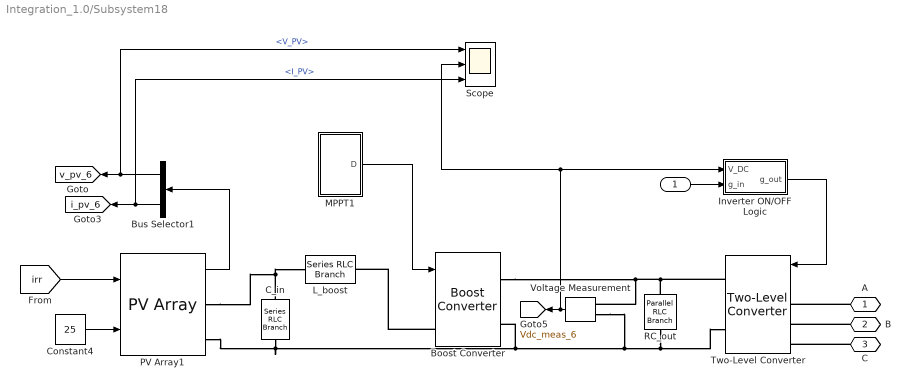
== system Integration_1.0/Subsystem18 ==
  "  " : Inport
  Boost Converter : spsBoostConverterLib/Boost Converter  ModelType=Average model (D-controlled)  Ron=1e-3  Rs=1e6  Cs=inf  Vforward=[0,0]  Ron_Diode=1e-3  Rs_Diode=1e6  Cs_Diode=inf  Vf_Diode=1e-3  Rs_CurrentSource=inf  Ron_ACsource=1e-3
      settings: LibrarySourceBlock=sps_lib/Power Electronics/Boost Converter
  Bus Selector1 : BusSelector  OutputSignals=V_PV,I_PV
  C_in : spsSeriesRLCBranchLib/Series RLC Branch  LConnTagsString=__new0  RConnTagsString=__new0  BranchType=C  Resistance=1e-5  Inductance=1e-3  SetiL0=off  InitialCurrent=0  Capacitance=1.5*241.03e-6  Setx0=off  InitialVoltage=426.5  Measurements=Branch voltage and current
  Constant4 : Constant  Value=25
  Inverter ON/OFF Logic : Subsystem
  L_boost : spsSeriesRLCBranchLib/Series RLC Branch  LConnTagsString=__new0  RConnTagsString=__new0  BranchType=L  Resistance=1e-3  Inductance=100e-3  SetiL0=off  InitialCurrent=0  Capacitance=100e-6  Setx0=off  InitialVoltage=230  Measurements=None
  MPPT1 : Subsystem
  PV Array1 : spsPVArrayLib/PV Array  Npar=4  Nser=6  PlotType=array @ 1000 W/m2 & specified temperatures  S_vec="[ 1000  500  100 ]"  Temp_C_vec="[ 45 25  ]"  ModuleName=SunPower SPR-415E-WHT-D  PlotWhenSelected=off  Pm=414.801  Ncell=128  Voc=85.3  Isc=6.09  Vm=72.9  Im=5.69  beta_Voc_pc=-0.229  alpha_Isc_pc=0.030706  beta_Voc=-0.19534  alpha_Isc=0.00187  IL=6.0978  I0=7.1698e-13  nI=0.87223  Rsh=419.7781  Rs=0.53711  RobustModel=off  RobustCellTemperature=313.3991  BAL=on  Tc=1e-6  Tfilter=5e-5
  RC_out : spsParallelRLCBranchLib/Parallel RLC Branch  LConnTagsString=a  RConnTagsString=__new0  BranchType=C  Resistance=5  Inductance=1e-3  SetiL0=off  InitialCurrent=0  Capacitance=5*220e-6  Setx0=off  InitialVoltage=700  Measurements=None
  Scope : Scope  NumInputPorts=3
  Two-Level Converter : spsTwoLevelConverterLib/Two-Level Converter  ModelType=Average model (No rectifier mode)  Ron=1e-3  Rs=1e6  Cs=inf  Vforward=[0,0]  Ron_Diode=1e-3  Rs_Diode=1e6  Cs_Diode=inf  Vf_Diode=1e-3  Rs_CurrentSource=inf  Ron_ACsource=1e-3
  Voltage Measurement : spsVoltageMeasurementLib/Voltage Measurement  PhasorSimulation=off  OutputType=Complex  PSBequivalent=0
  A : PMIOPort  Side=Left
  B : PMIOPort  Port=2  Side=Left
  C : PMIOPort  Port=3  Side=Left
  tag scope: Vdc_meas_6=global, i_pv_6=global, v_pv_6=global
  wires:
  Bus Selector1/1 -> Scope/1, [v_pv_6]  "<V_PV>"
  Constant4/1 -> PV Array1/2
  Bus Selector1/2 -> Scope/3, [i_pv_6]  "<I_PV>"
  PV Array1/1 -> Bus Selector1/1
  [irr] -> PV Array1/1
  Inverter ON/OFF Logic/1(g_out) -> Two-Level Converter/1
  MPPT1/1(D) -> Boost Converter/1
  Voltage Measurement/1 -> Inverter ON/OFF Logic/1(V_DC), Scope/2, [Vdc_meas_6]
  "  "/1 -> Inverter ON/OFF Logic/2(g_in)
  connections:
  A/RConn1 -- Two-Level Converter/LConn1
  Two-Level Converter/RConn2 -- RC_out/RConn1 -- Voltage Measurement/LConn2 -- C_in/RConn1 -- PV Array1/RConn2 -- Boost Converter/RConn2
  C_in/LConn1 -- L_boost/LConn1 -- PV Array1/RConn1
  RC_out/LConn1 -- Boost Converter/RConn1 -- Voltage Measurement/LConn1 -- Two-Level Converter/RConn1
  C/RConn1 -- Two-Level Converter/LConn3
  B/RConn1 -- Two-Level Converter/LConn2
  Boost Converter/LConn1 -- L_boost/RConn1

== system Integration_1.0/Subsystem19 ==
  Ground1 : spsGroundLib/Ground  LConnTagsString=a
  Subsystem2 : Subsystem
  A : PMIOPort  Side=Left
  B : PMIOPort  Port=2  Side=Left
  C : PMIOPort  Port=3  Side=Left
  connections:
  Subsystem2/LConn2 -- B/RConn1
  Subsystem2/LConn4 -- Ground1/LConn1
  Subsystem2/LConn1 -- A/RConn1
  Subsystem2/LConn3 -- C/RConn1

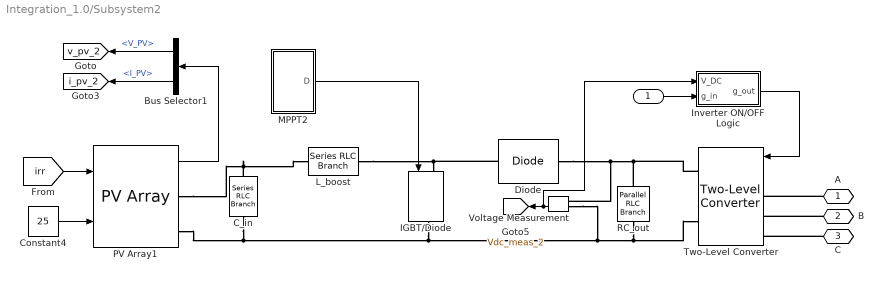
== system Integration_1.0/Subsystem2 ==
  "  " : Inport
  Bus Selector1 : BusSelector  OutputSignals=V_PV,I_PV
  C_in : spsSeriesRLCBranchLib/Series RLC Branch  LConnTagsString=__new0  RConnTagsString=__new0  BranchType=C  Resistance=1e-5  Inductance=1e-3  SetiL0=off  InitialCurrent=0  Capacitance=3029e-6  Setx0=off  InitialVoltage=426.5  Measurements=Branch voltage and current
  Constant4 : Constant  Value=25
  Diode : spsDiodeLib/Diode  Ron=0.001  Lon=0  Vf=0.8  IC=0  UseSnubber=0  Rs=500  Cs=250e-9  Measurements=off
  IGBT/Diode : spsIGBTDiodeLib/IGBT//Diode  Ron=1e-3  Rs=1e5  Cs=inf  Measurements=off
  Inverter ON/OFF Logic : Subsystem
  L_boost : spsSeriesRLCBranchLib/Series RLC Branch  LConnTagsString=__new0  RConnTagsString=__new0  BranchType=L  Resistance=1e-3  Inductance=60e-3  SetiL0=off  InitialCurrent=0  Capacitance=100e-6  Setx0=off  InitialVoltage=230  Measurements=None
  MPPT2 : Subsystem
  PV Array1 : spsPVArrayLib/PV Array  Npar=2  Nser=5  PlotType=array @ 1000 W/m2 & specified temperatures  S_vec="[ 1000  500  100 ]"  Temp_C_vec="[ 45 25  ]"  ModuleName=SunPower SPR-415E-WHT-D  PlotWhenSelected=off  Pm=414.801  Ncell=128  Voc=85.3  Isc=6.09  Vm=72.9  Im=5.69  beta_Voc_pc=-0.229  alpha_Isc_pc=0.030706  beta_Voc=-0.19534  alpha_Isc=0.00187  IL=6.0978  I0=7.1698e-13  nI=0.87223  Rsh=419.7781  Rs=0.53711  RobustModel=off  RobustCellTemperature=313.3991  BAL=on  Tc=1e-6  Tfilter=5e-5
  RC_out : spsParallelRLCBranchLib/Parallel RLC Branch  LConnTagsString=a  RConnTagsString=__new0  BranchType=C  Resistance=5  Inductance=1e-3  SetiL0=off  InitialCurrent=0  Capacitance=5*922e-6  Setx0=off  InitialVoltage=700  Measurements=None
  Two-Level Converter : spsTwoLevelConverterLib/Two-Level Converter  ModelType=Average model (No rectifier mode)  Ron=1e-3  Rs=1e6  Cs=inf  Vforward=[0,0]  Ron_Diode=1e-3  Rs_Diode=1e6  Cs_Diode=inf  Vf_Diode=1e-3  Rs_CurrentSource=inf  Ron_ACsource=1e-3
  Voltage Measurement : spsVoltageMeasurementLib/Voltage Measurement  PhasorSimulation=off  OutputType=Complex  PSBequivalent=0
  A : PMIOPort  Side=Left
  B : PMIOPort  Port=2  Side=Left
  C : PMIOPort  Port=3  Side=Left
  tag scope: Vdc_meas_2=global, i_pv_2=global, v_pv_2=global
  wires:
  Voltage Measurement/1 -> Inverter ON/OFF Logic/1(V_DC), [Vdc_meas_2]
  Bus Selector1/1 -> [v_pv_2]  "<V_PV>"
  Constant4/1 -> PV Array1/2
  Bus Selector1/2 -> [i_pv_2]  "<I_PV>"
  PV Array1/1 -> Bus Selector1/1
  MPPT2/1(D) -> IGBT/Diode/1
  [irr] -> PV Array1/1
  Inverter ON/OFF Logic/1(g_out) -> Two-Level Converter/1
  "  "/1 -> Inverter ON/OFF Logic/2(g_in)
  connections:
  A/RConn1 -- Two-Level Converter/LConn1
  Two-Level Converter/RConn2 -- RC_out/RConn1 -- IGBT/Diode/RConn1 -- C_in/RConn1 -- PV Array1/RConn2 -- Voltage Measurement/LConn2
  C_in/LConn1 -- L_boost/LConn1 -- PV Array1/RConn1
  RC_out/LConn1 -- Two-Level Converter/RConn1 -- Diode/RConn1 -- Voltage Measurement/LConn1
  C/RConn1 -- Two-Level Converter/LConn3
  B/RConn1 -- Two-Level Converter/LConn2
  L_boost/RConn1 -- Diode/LConn1 -- IGBT/Diode/LConn1

== system Integration_1.0/Subsystem3 ==
  Series RLC Branch1 : spsSeriesRLCBranchLib/Series RLC Branch  LConnTagsString=__new0  RConnTagsString=__new0  BranchType=RC  Resistance=10  Inductance=1e-3  SetiL0=off  InitialCurrent=0  Capacitance=1.316e-6  Setx0=off  InitialVoltage=0  Measurements=None
  Series RLC Branch2 : spsSeriesRLCBranchLib/Series RLC Branch  LConnTagsString=__new0  RConnTagsString=__new0  BranchType=RC  Resistance=10  Inductance=1e-3  SetiL0=off  InitialCurrent=0  Capacitance=1.316e-6  Setx0=off  InitialVoltage=0  Measurements=None
  Series RLC Branch3 : spsSeriesRLCBranchLib/Series RLC Branch  LConnTagsString=__new0  RConnTagsString=__new0  BranchType=RC  Resistance=10  Inductance=1e-3  SetiL0=off  InitialCurrent=0  Capacitance=1.316e-6  Setx0=off  InitialVoltage=0  Measurements=None
  Three-Phase Series RLC Branch1 : spsThreePhaseSeriesRLCBranchLib/Three-Phase Series RLC Branch  LConnTagsString=A|B|C  RConnTagsString=A|B|C  BranchType=L  Resistance=1  Inductance=3*2.309e-3  Capacitance=1e-6  Measurements=None
  A : PMIOPort  Side=Left
  B : PMIOPort  Port=2  Side=Left
  C : PMIOPort  Port=3  Side=Left
  a : PMIOPort  Port=4  Side=Right
  b : PMIOPort  Port=5  Side=Right
  c : PMIOPort  Port=6  Side=Right
  connections:
  Series RLC Branch1/LConn1 -- Three-Phase Series RLC Branch1/RConn2 -- b/RConn1 -- Series RLC Branch3/RConn1
  Series RLC Branch3/LConn1 -- a/RConn1 -- Three-Phase Series RLC Branch1/RConn1 -- Series RLC Branch2/RConn1
  Three-Phase Series RLC Branch1/LConn1 -- A/RConn1
  Three-Phase Series RLC Branch1/LConn2 -- B/RConn1
  Three-Phase Series RLC Branch1/LConn3 -- C/RConn1
  Three-Phase Series RLC Branch1/RConn3 -- c/RConn1 -- Series RLC Branch1/RConn1 -- Series RLC Branch2/LConn1

== system Integration_1.0/Subsystem4 ==
  Ground1 : spsGroundLib/Ground  LConnTagsString=a
  Subsystem2 : Subsystem
  A : PMIOPort  Side=Left
  B : PMIOPort  Port=2  Side=Left
  C : PMIOPort  Port=3  Side=Left
  connections:
  Subsystem2/LConn2 -- B/RConn1
  Subsystem2/LConn4 -- Ground1/LConn1
  Subsystem2/LConn1 -- A/RConn1
  Subsystem2/LConn3 -- C/RConn1

== system Integration_1.0/Subsystem5 ==
  Ground : spsGroundLib/Ground  LConnTagsString=a
  "Grounding Transformer " : spsGroundingTransformerLib/Grounding Transformer   UNITS=SI  NominalPower="[3e3   50]"  NominalVoltage=0.4e3  ZeroSequenceImpedance_pu=[0.025 0.75]  MagnetizationBranch_pu=[500 500]  ZeroSequenceImpedance_SI=[1.3333 40]  MagnetizationBranch_SI=[26667 26667]  Measurements=All voltages and currents
      settings: LibrarySourceBlock=|
      | sps_lib/Power Grid Elements/Grounding
      | Transformer
  Three-Phase Series RLC Branch1 : spsThreePhaseSeriesRLCBranchLib/Three-Phase Series RLC Branch  Commented=on  LConnTagsString=A|B|C  RConnTagsString=A|B|C  BranchType=RL  Resistance=0.02  Inductance=3e-3  Capacitance=1e-6  Measurements=None
  Three-Phase Source : spsThreePhaseSourceLib/Three-Phase Source  InternalConnection=Yg  VoltagePhases=off  Voltage=400  PhaseAngle=0  Voltage_phases=[25e3 25e3 25e3]/sqrt(3)  PhaseAngles_phases=[0 -120 +120]  Frequency=50  NonIdealSource=on  SpecifyImpedance=on  Resistance=0.0113  Inductance=36e-6  ShortCircuitLevel=10e6  BaseVoltage=400  XRratio=5  BusType=swing  Pref=10e3  Qref=0  Prefabc=[10e3, 10e3, 10e3]  Qrefabc=[0, 0, 0]  Qmin=-inf  Qmax=inf
  A : PMIOPort  Side=Left
  B : PMIOPort  Port=2  Side=Left
  C : PMIOPort  Port=3  Side=Left
  connections:
  "Grounding Transformer "/RConn1 -- Ground/LConn1
  A/RConn1 -- "Grounding Transformer "/LConn1 -- Three-Phase Source/RConn1
  "Grounding Transformer "/LConn3 -- Three-Phase Source/RConn3 -- C/RConn1
  "Grounding Transformer "/LConn2 -- B/RConn1 -- Three-Phase Source/RConn2

== system Integration_1.0/Subsystem6 ==
  Ground1 : spsGroundLib/Ground  LConnTagsString=a
  Subsystem2 : Subsystem
  A : PMIOPort  Side=Left
  B : PMIOPort  Port=2  Side=Left
  C : PMIOPort  Port=3  Side=Left
  connections:
  Subsystem2/LConn2 -- B/RConn1
  Subsystem2/LConn4 -- Ground1/LConn1
  Subsystem2/LConn1 -- A/RConn1
  Subsystem2/LConn3 -- C/RConn1

== system Integration_1.0/Subsystem7 ==
  Ground1 : spsGroundLib/Ground  LConnTagsString=a
  Subsystem2 : Subsystem
  A : PMIOPort  Side=Left
  B : PMIOPort  Port=2  Side=Left
  C : PMIOPort  Port=3  Side=Left
  connections:
  Subsystem2/LConn2 -- B/RConn1
  Subsystem2/LConn4 -- Ground1/LConn1
  Subsystem2/LConn1 -- A/RConn1
  Subsystem2/LConn3 -- C/RConn1

== system Integration_1.0/Subsystem8 ==
  Series RLC Branch1 : spsSeriesRLCBranchLib/Series RLC Branch  LConnTagsString=__new0  RConnTagsString=__new0  BranchType=C  Resistance=5  Inductance=1e-3  SetiL0=off  InitialCurrent=0  Capacitance=0.322e-6  Setx0=off  InitialVoltage=0  Measurements=None
  Series RLC Branch2 : spsSeriesRLCBranchLib/Series RLC Branch  LConnTagsString=__new0  RConnTagsString=__new0  BranchType=C  Resistance=5  Inductance=1e-3  SetiL0=off  InitialCurrent=0  Capacitance=0.322e-6  Setx0=off  InitialVoltage=0  Measurements=None
  Series RLC Branch3 : spsSeriesRLCBranchLib/Series RLC Branch  LConnTagsString=__new0  RConnTagsString=__new0  BranchType=C  Resistance=5  Inductance=1e-3  SetiL0=off  InitialCurrent=0  Capacitance=0.322e-6  Setx0=off  InitialVoltage=0  Measurements=None
  Three-Phase Series RLC Branch1 : spsThreePhaseSeriesRLCBranchLib/Three-Phase Series RLC Branch  LConnTagsString=A|B|C  RConnTagsString=A|B|C  BranchType=L  Resistance=1  Inductance=3*9.42e-3  Capacitance=1e-6  Measurements=None
  A : PMIOPort  Side=Left
  B : PMIOPort  Port=2  Side=Left
  C : PMIOPort  Port=3  Side=Left
  a : PMIOPort  Port=4  Side=Right
  b : PMIOPort  Port=5  Side=Right
  c : PMIOPort  Port=6  Side=Right
  connections:
  c/RConn1 -- Three-Phase Series RLC Branch1/RConn3 -- Series RLC Branch2/LConn1 -- Series RLC Branch1/RConn1
  Three-Phase Series RLC Branch1/LConn3 -- C/RConn1
  Three-Phase Series RLC Branch1/LConn2 -- B/RConn1
  Three-Phase Series RLC Branch1/LConn1 -- A/RConn1
  a/RConn1 -- Three-Phase Series RLC Branch1/RConn1 -- Series RLC Branch3/LConn1 -- Series RLC Branch2/RConn1
  b/RConn1 -- Series RLC Branch3/RConn1 -- Series RLC Branch1/LConn1 -- Three-Phase Series RLC Branch1/RConn2

== system Integration_1.0/Subsystem9 ==
  "  " : Inport
  Boost Converter : spsBoostConverterLib/Boost Converter  ModelType=Average model (D-controlled)  Ron=1e-3  Rs=1e6  Cs=inf  Vforward=[0,0]  Ron_Diode=1e-3  Rs_Diode=1e6  Cs_Diode=inf  Vf_Diode=1e-3  Rs_CurrentSource=inf  Ron_ACsource=1e-3
      settings: LibrarySourceBlock=sps_lib/Power Electronics/Boost Converter
  Bus Selector1 : BusSelector  OutputSignals=V_PV,I_PV
  C_in : spsSeriesRLCBranchLib/Series RLC Branch  LConnTagsString=__new0  RConnTagsString=__new0  BranchType=C  Resistance=1e-5  Inductance=1e-3  SetiL0=off  InitialCurrent=0  Capacitance=314e-6  Setx0=off  InitialVoltage=426.5  Measurements=Branch voltage and current
  Constant4 : Constant  Value=25
  Inverter ON/OFF Logic : Subsystem
  L_boost : spsSeriesRLCBranchLib/Series RLC Branch  LConnTagsString=__new0  RConnTagsString=__new0  BranchType=L  Resistance=1e-3  Inductance=157e-3  SetiL0=off  InitialCurrent=0  Capacitance=100e-6  Setx0=off  InitialVoltage=230  Measurements=None
  MPPT2 : Subsystem
  PV Array1 : spsPVArrayLib/PV Array  Npar=3  Nser=5  PlotType=array @ 1000 W/m2 & specified temperatures  S_vec="[ 1000  500  100 ]"  Temp_C_vec="[ 45 25  ]"  ModuleName=SunPower SPR-415E-WHT-D  PlotWhenSelected=off  Pm=414.801  Ncell=128  Voc=85.3  Isc=6.09  Vm=72.9  Im=5.69  beta_Voc_pc=-0.229  alpha_Isc_pc=0.030706  beta_Voc=-0.19534  alpha_Isc=0.00187  IL=6.0978  I0=7.1698e-13  nI=0.87223  Rsh=419.7781  Rs=0.53711  RobustModel=off  RobustCellTemperature=313.3991  BAL=on  Tc=1e-6  Tfilter=5e-5
  RC_out : spsParallelRLCBranchLib/Parallel RLC Branch  LConnTagsString=a  RConnTagsString=__new0  BranchType=C  Resistance=5  Inductance=1e-3  SetiL0=off  InitialCurrent=0  Capacitance=5*239e-6  Setx0=off  InitialVoltage=700  Measurements=None
  Two-Level Converter : spsTwoLevelConverterLib/Two-Level Converter  ModelType=Average model (No rectifier mode)  Ron=1e-3  Rs=1e6  Cs=inf  Vforward=[0,0]  Ron_Diode=1e-3  Rs_Diode=1e6  Cs_Diode=inf  Vf_Diode=1e-3  Rs_CurrentSource=inf  Ron_ACsource=1e-3
  Voltage Measurement : spsVoltageMeasurementLib/Voltage Measurement  PhasorSimulation=off  OutputType=Complex  PSBequivalent=0
  A : PMIOPort  Side=Left
  B : PMIOPort  Port=2  Side=Left
  C : PMIOPort  Port=3  Side=Left
  tag scope: Vdc_meas_3=global, i_pv_3=global, v_pv_3=global
  wires:
  Bus Selector1/1 -> [v_pv_3]  "<V_PV>"
  Constant4/1 -> PV Array1/2
  Bus Selector1/2 -> [i_pv_3]  "<I_PV>"
  PV Array1/1 -> Bus Selector1/1
  [irr] -> PV Array1/1
  MPPT2/1(D) -> Boost Converter/1
  Inverter ON/OFF Logic/1(g_out) -> Two-Level Converter/1
  "  "/1 -> Inverter ON/OFF Logic/2(g_in)
  Voltage Measurement/1 -> Inverter ON/OFF Logic/1(V_DC), [Vdc_meas_3]
  connections:
  A/RConn1 -- Two-Level Converter/LConn1
  Two-Level Converter/RConn2 -- RC_out/RConn1 -- Voltage Measurement/LConn2 -- Boost Converter/RConn2 -- C_in/RConn1 -- PV Array1/RConn2
  C_in/LConn1 -- L_boost/LConn1 -- PV Array1/RConn1
  RC_out/LConn1 -- Two-Level Converter/RConn1 -- Boost Converter/RConn1 -- Voltage Measurement/LConn1
  C/RConn1 -- Two-Level Converter/LConn3
  B/RConn1 -- Two-Level Converter/LConn2
  L_boost/RConn1 -- Boost Converter/LConn1
